simulink model "dsp_proj_v1"  (R2024b)
settings: Solver=VariableStepAuto  StartTime=0.0  StopTime=10.0  RelTol=1e-3
libraries: hdlsllib x9, simulink x4
settings Model: Creator=UTSAB KARAN  LastModifiedBy=UTSAB KARAN

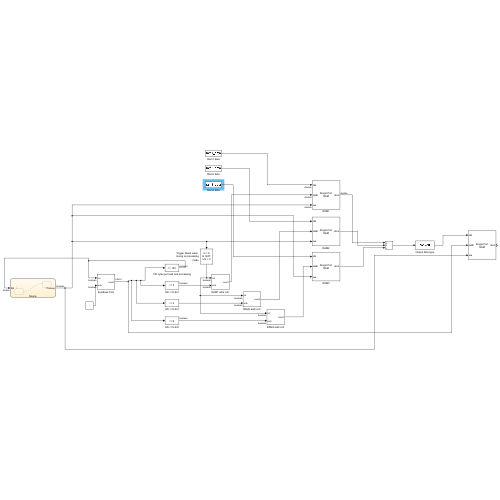
[thumbnail: Simulink's stored preview of the top-level diagram]
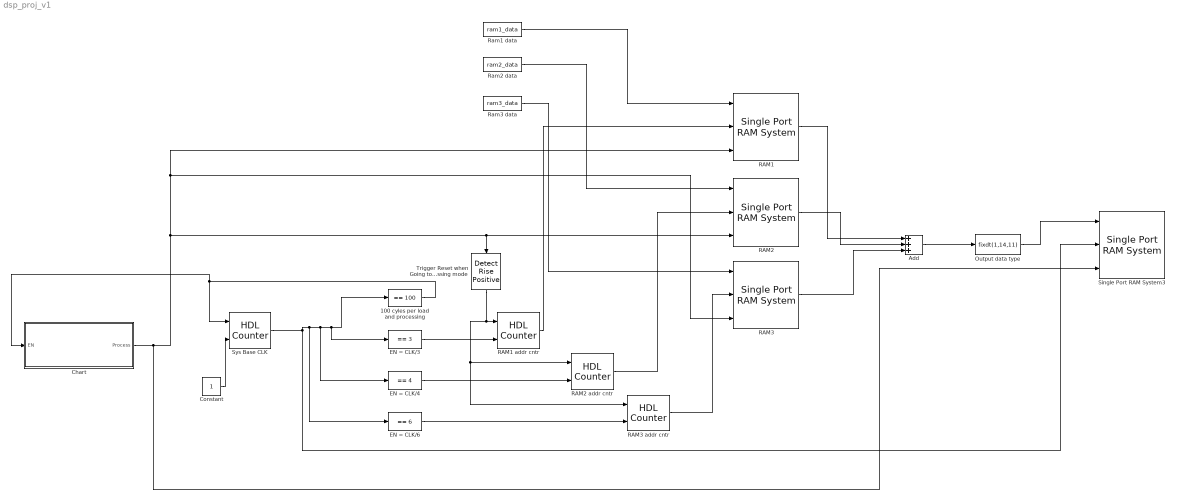
== system dsp_proj_v1 ==
  100 cyles per load and processing : simulink/Logic and Bit Operations/Compare To Constant  relop===  const=100  OutDataTypeStr=boolean
  Add : Sum  Inputs=+++
  Chart : Stateflow chart  TreatAsAtomicUnit=on
  Constant : Constant
  EN = CLK/3 : simulink/Logic and Bit Operations/Compare To Constant  relop===  const=3  OutDataTypeStr=boolean
  EN = CLK/4 : simulink/Logic and Bit Operations/Compare To Constant  relop===  const=4  OutDataTypeStr=boolean
  EN = CLK/6 : simulink/Logic and Bit Operations/Compare To Constant  relop===  const=6  OutDataTypeStr=boolean
  Output data type : DataTypeConversion  OutDataTypeStr=fixdt(1,14,11)  SaturateOnIntegerOverflow=off  RndMeth=Floor  LockScale=on
  RAM1 : hdlsllib/HDL RAMs/Single Port RAM System  RAMType=Single port  AsyncRead=off  WriteOutputValue=New data  RAMInitialValue=0  allowBusInputs=off  WritesHaveOutput=on  NumReads=0  NumWrites=1  SimulateUsing=Code generation  ModelRAMDelay=on
  RAM1 addr cntr : hdlsllib/Sources/HDL Counter  CountType=Count limited  CountInit=0  CountStep=1  CountMax=1000  CountFromType=Initial value  CountFrom=0  CountResetPort=on  CountLoadPort=off  CountEnbPort=on  CountDirPort=off  CountHitOutputPort=off  CountDataType=Unsigned  CountWordLen=12  CountFracLen=0  CountSampTime=1
  RAM2 : hdlsllib/HDL RAMs/Single Port RAM System  RAMType=Single port  AsyncRead=off  WriteOutputValue=New data  RAMInitialValue=0  allowBusInputs=off  WritesHaveOutput=on  NumReads=0  NumWrites=1  SimulateUsing=Code generation  ModelRAMDelay=on
  RAM2 addr cntr : hdlsllib/Sources/HDL Counter  CountType=Count limited  CountInit=0  CountStep=1  CountMax=1000  CountFromType=Initial value  CountFrom=0  CountResetPort=on  CountLoadPort=off  CountEnbPort=on  CountDirPort=off  CountHitOutputPort=off  CountDataType=Unsigned  CountWordLen=12  CountFracLen=0  CountSampTime=1
  RAM3 : hdlsllib/HDL RAMs/Single Port RAM System  RAMType=Single port  AsyncRead=off  WriteOutputValue=New data  RAMInitialValue=0  allowBusInputs=off  WritesHaveOutput=on  NumReads=0  NumWrites=1  SimulateUsing=Code generation  ModelRAMDelay=on
  RAM3 addr cntr : hdlsllib/Sources/HDL Counter  CountType=Count limited  CountInit=0  CountStep=1  CountMax=1000  CountFromType=Initial value  CountFrom=0  CountResetPort=on  CountLoadPort=off  CountEnbPort=on  CountDirPort=off  CountHitOutputPort=off  CountDataType=Unsigned  CountWordLen=12  CountFracLen=0  CountSampTime=1
  Ram1 data : FromWorkspace  VariableName=ram1_data
  Ram2 data : FromWorkspace  VariableName=ram2_data
  Ram3 data : FromWorkspace  VariableName=ram3_data
  Single Port RAM System3 : hdlsllib/HDL RAMs/Single Port RAM System  RAMType=Single port  AsyncRead=off  WriteOutputValue=New data  RAMInitialValue=0  allowBusInputs=off  WritesHaveOutput=on  NumReads=0  NumWrites=1  SimulateUsing=Code generation  ModelRAMDelay=on
  Sys Base CLK : hdlsllib/Sources/HDL Counter  CountType=Count limited  CountInit=0  CountStep=1  CountMax=1000  CountFromType=Initial value  CountFrom=0  CountResetPort=on  CountLoadPort=off  CountEnbPort=on  CountDirPort=off  CountHitOutputPort=off  CountDataType=Unsigned  CountWordLen=12  CountFracLen=0  CountSampTime=1
  Trigger Reset when Going to processing mode : hdlsllib/Logic and Bit Operations/Detect Rise Positive  vinit=0  OutDataTypeStr=boolean
  wires:
  Sys Base CLK/1 -> EN = CLK/6/1, EN = CLK/4/1, EN = CLK/3/1, 100 cyles per load and processing/1, Single Port RAM System3/2
  Constant/1 -> Sys Base CLK/2
  100 cyles per load and processing/1 -> Chart/1(EN), Sys Base CLK/1
  EN = CLK/3/1 -> RAM1 addr cntr/2
  EN = CLK/4/1 -> RAM2 addr cntr/2
  EN = CLK/6/1 -> RAM3 addr cntr/2
  RAM1 addr cntr/1 -> RAM1/2
  RAM2 addr cntr/1 -> RAM2/2
  RAM3 addr cntr/1 -> RAM3/2
  RAM2/1 -> Add/2
  RAM3/1 -> Add/3
  RAM1/1 -> Add/1
  Add/1 -> Output data type/1
  Output data type/1 -> Single Port RAM System3/1
  Chart/1(Process) -> Single Port RAM System3/3, RAM1/3, RAM3/3, Trigger Reset when Going to processing mode/1, RAM2/3
  Ram1 data/1 -> RAM1/1
  Ram2 data/1 -> RAM2/1
  Ram3 data/1 -> RAM3/1
  Trigger Reset when Going to processing mode/1 -> RAM3 addr cntr/1, RAM2 addr cntr/1, RAM1 addr cntr/1

== stateflow chart dsp_proj_v1/Chart ==
  settings: stateMachineType=MOORE_MACHINE  executeAtInitialization=1
  state Processing
    Process = true
  state Data_Loading
    Process = false
  Data_Loading -> Processing : [ EN==1]
  (default) -> Data_Loading
  data: Process output; EN input
